simulink model "fz6_5"  (R2014a)
settings: Solver=ode45  StartTime=0.0  StopTime=100000  RelTol=1e-3
libraries: commsink2 x1, commchan3 x1, dspmathops x1, commrandsrc2 x1
settings Model: Creator=tzb  LastModifiedBy=tzb

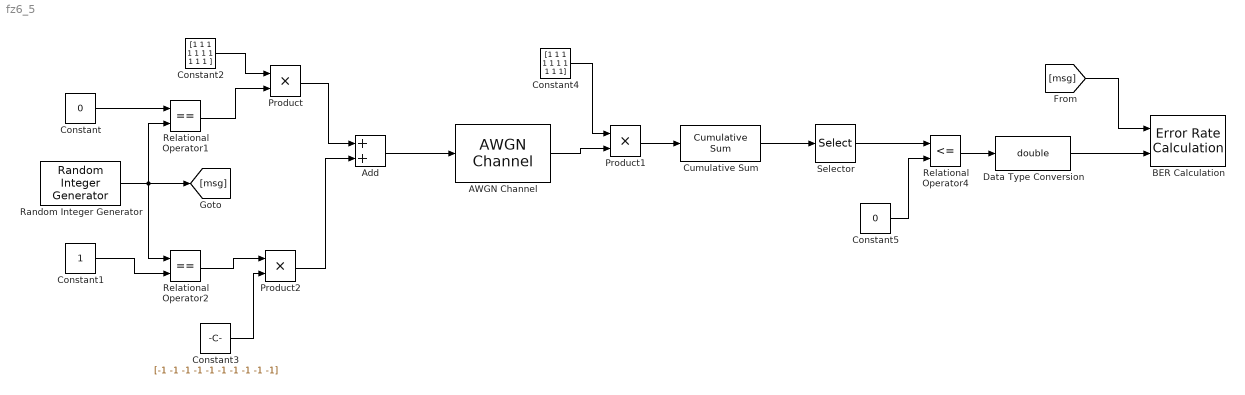
== system fz6_5 ==
  " BER Calculation" : commsink2/Error Rate Calculation  N=0  st_delay=0  cp_mode=Entire frame  subframe=[]  PMode=Workspace  WsName=BER  RsMode2=off  stop=off  numErr=100  maxBits=1e6
  AWGN Channel : commchan3/AWGN Channel  InputProcessing=Inherited (this choice will be removed - see release notes)  seed=67  noiseMode="Signal to noise ratio  (Eb/No)"  EbNodB=SNR  EsNodB=10  SNRdB=10  bitsPerSym=1  Ps=1  Tsym=1  variance=1
  Add : Sum
  Constant : Constant  Value=0
  Constant1 : Constant
  Constant2 : Constant  Value=[1 1 1 1 1 1 1 1 1 1 ]  SampleTime=0.1
  Constant3 : Constant  Value=[-1 -1 -1 -1 -1 -1 -1 -1 -1 -1]  SampleTime=0.1
  Constant4 : Constant  Value=[1 1 1 1 1 1 1 1 1 1]
  Constant5 : Constant  Value=0
  Cumulative Sum : dspmathops/Cumulative Sum  dim=Rows  InputProcessing=Columns as channels (frame based)  reset_popup=None  outputDataTypeStr=Inherit: Same as accumulator  outputLastDataTypeStr=Inherit: Same as accumulator  outputMin=[]  outputMax=[]  roundingMode=Floor  overflowMode=off
  Data Type Conversion : DataTypeConversion  OutDataTypeStr=double
  Product : Product
  Product1 : Product
  Product2 : Product
  Random Integer Generator : commrandsrc2/Random Integer Generator  mul=2  seed=1234  Ts=1  frameBased=off  sampPerFrame=1  orient=off  outDataType=double
  Relational Operator1 : RelationalOperator  Operator===  OutDataTypeStr=boolean
  Relational Operator2 : RelationalOperator  Operator===  OutDataTypeStr=boolean
  Relational Operator4 : RelationalOperator  Operator=<=  OutDataTypeStr=boolean
  Selector : Selector  InputPortWidth=10  Indices=[10]
  wires:
  Selector/1 -> Relational Operator4/1
  Random Integer Generator/1 -> Relational Operator1/2, Relational Operator2/1, [msg]
  Constant/1 -> Relational Operator1/1
  Constant1/1 -> Relational Operator2/2
  Relational Operator2/1 -> Product2/1
  Constant3/1 -> Product2/2
  Relational Operator1/1 -> Product/2
  Constant2/1 -> Product/1
  Product/1 -> Add/1
  Product2/1 -> Add/2
  Add/1 -> AWGN Channel/1
  AWGN Channel/1 -> Product1/2
  Constant4/1 -> Product1/1
  Product1/1 -> Cumulative Sum/1
  Cumulative Sum/1 -> Selector/1
  Constant5/1 -> Relational Operator4/2
  Relational Operator4/1 -> Data Type Conversion/1
  [msg] -> " BER Calculation"/1
  Data Type Conversion/1 -> " BER Calculation"/2
